simulink model "ejemp_fullp"  (Simulink 8.4)
settings: Solver=ode45  StartTime=0.0  StopTime=length(a)  RelTol=1e-3
libraries: dspsrcs4 x3
settings Model: Creator=jvalls  LastModifiedBy=jvalls
settings DataIOCC: SignalLoggingSaveFormat=Dataset
settings OptimizationCC: ExpressionDepthLimit=128
settings DebuggingCC: UnderspecifiedInitializationDetection=Simplified  MergeDetectMultiDrivingBlocksExec=error  FcnCallInpInsideContextMsg=EnableAllAsError  StateNameClashWarn=none
settings GRTTargetCC: CombineOutputUpdateFcns=on  GRTInterface=off

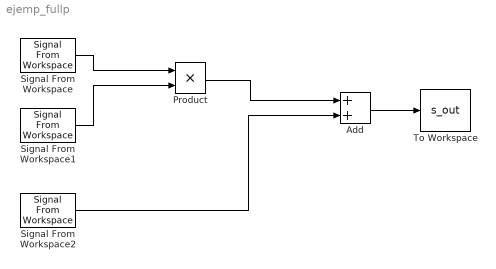
== system ejemp_fullp ==
  Add : Sum  AccumDataTypeStr=double  OutDataTypeStr=double
  Product : Product  OutDataTypeStr=double
  Signal From Workspace : dspsrcs4/Signal From Workspace  X=a  Ts=1  nsamps=1  OutputAfterFinalValue=Setting to zero  ignoreOrWarnInputAndFrameLengths=off
  Signal From Workspace1 : dspsrcs4/Signal From Workspace  X=b  Ts=1  nsamps=1  OutputAfterFinalValue=Setting to zero  ignoreOrWarnInputAndFrameLengths=off
  Signal From Workspace2 : dspsrcs4/Signal From Workspace  X=c  Ts=1  nsamps=1  OutputAfterFinalValue=Setting to zero  ignoreOrWarnInputAndFrameLengths=off
  To Workspace : ToWorkspace  VariableName=s_out  SampleTime=-1
      settings: Save2DSignal=2-D array (concatenate along first dimension)
  wires:
  Product/1 -> Add/1
  Signal From Workspace/1 -> Product/1
  Signal From Workspace1/1 -> Product/2
  Signal From Workspace2/1 -> Add/2
  Add/1 -> To Workspace/1
